simulink model "test_environment"  (R2019b)
settings: Solver=VariableStepAuto  StartTime=0.0  StopTime=100.0  FixedStep=1e-3  RelTol=1e-3
InitFcn:
  | data
undefined symbols (not defined in the file): __PRM__SERIALIZED__DATA__, juliandate, r, r_bo, RP, SubsystemReferenceBlock
libraries: simulink x4
settings Model: Creator=imanol  LastModifiedBy=imanol

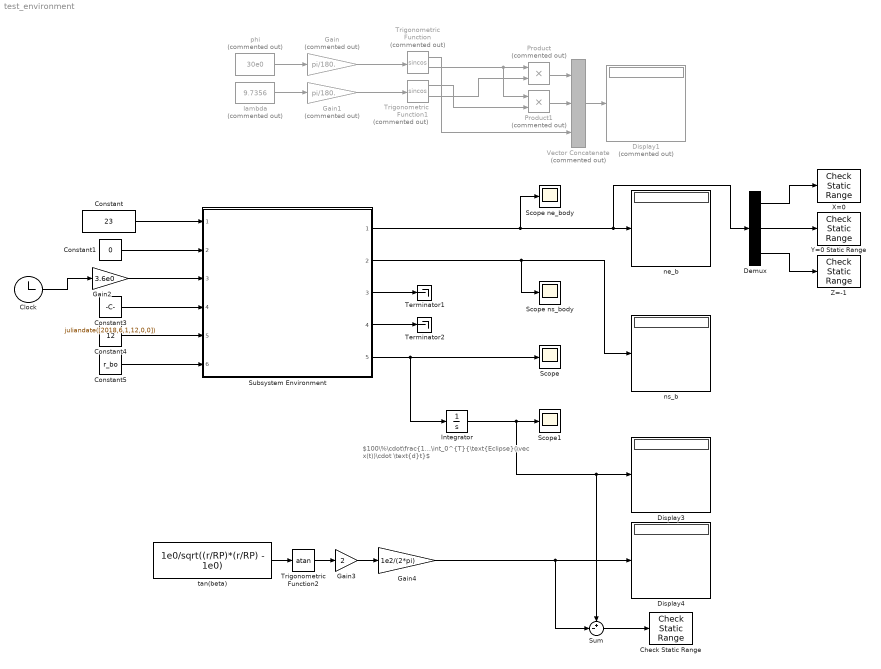
== system test_environment ==
  note: $100\%\cdot\frac{1}{T}\int_0^{T}{\text{Eclipse}(\vec x(t))\cdot \text{d}t}$
  Check Static Range : simulink/Model Verification/Check  Static Range  Description=-1e2 <= u <= 2e0  max=2e0  max_included=on  min=-1e2  min_included=on  enabled=on  stopWhenAssertionFail=on  export=off  icon=graphic
      settings: SourceProductName=Simulink  SourceProductBaseCode=SL
  Clock : Clock
      settings: Decimation=100
  Constant : Constant  Value=23
  Constant1 : Constant  Value=0
  Constant3 : Constant  Value=juliandate([2018,6,1,12,0,0])
  Constant4 : Constant  Value=12
  Constant5 : Constant  Value=r_bo
  Demux : Demux  Outputs=3
  Display1 : Display  Commented=on
  Display3 : Display
  Display4 : Display
  Gain : Gain  Commented=on  Gain=pi/180.
  Gain1 : Gain  Commented=on  Gain=pi/180.
  Gain2 : Gain  Gain=3.6e0
  Gain3 : Gain  Gain=2
  Gain4 : Gain  Gain=1e2/(2*pi)
  Integrator : Integrator  InitialCondition=0e0
  Product : Product  Commented=on
  Product1 : Product  Commented=on
  Scope : Scope
  Scope ne_body : Scope
  Scope ns_body : Scope
  Scope1 : Scope
  Subsystem Environment : Subsystem  BlockKeywords=__PRM__SERIALIZED__DATA__:SubsystemReferenceBlock  ReferencedSubsystem=block_environment
  Sum : Sum  Inputs=+-|
  Terminator1 : Terminator
  Terminator2 : Terminator
  Trigonometric Function : Trigonometry  Commented=on  Operator=sincos
  Trigonometric Function1 : Trigonometry  Commented=on  Operator=sincos
  Trigonometric Function2 : Trigonometry  Operator=atan
  Vector Concatenate : Concatenate  Commented=on  NumInputs=3
  X=0 : simulink/Model Verification/Check  Static Range  Description=0e0 - 1e-5 <= u <= 0e0 + 1e-5  max=0e0 + 1e-5  max_included=on  min=0e0 - 1e-5  min_included=on  enabled=on  stopWhenAssertionFail=on  export=off  icon=graphic
      settings: SourceProductName=Simulink  SourceProductBaseCode=SL
  Y=0 Static Range : simulink/Model Verification/Check  Static Range  Description=0e0 - 1e-5 <= u <= 0e0 + 1e-5  max=0e0 + 1e-5  max_included=on  min=0e0 - 1e-5  min_included=on  enabled=on  stopWhenAssertionFail=on  export=off  icon=graphic
      settings: SourceProductName=Simulink  SourceProductBaseCode=SL
  "Z=-1 " : simulink/Model Verification/Check  Static Range  Description=-1e0 - 1e-5 <= u <= -1e0 + 1e-5  max=-1e0 + 1e-5  max_included=on  min=-1e0 - 1e-5  min_included=on  enabled=on  stopWhenAssertionFail=on  export=off  icon=graphic
      settings: SourceProductName=Simulink  SourceProductBaseCode=SL
  lambda : Constant  Commented=on  Value=9.7356
  ne_b : Display
  ns_b : Display
  phi : Constant  Commented=on  Value=30e0
  tan(beta) : Constant  Value=1e0/sqrt((r/RP)*(r/RP) - 1e0)
  wires:
  Constant/1 -> Subsystem Environment/1
  Constant1/1 -> Subsystem Environment/2
  Gain2/1 -> Subsystem Environment/3
  Constant3/1 -> Subsystem Environment/4
  Constant4/1 -> Subsystem Environment/5
  Subsystem Environment/1 -> Scope ne_body/1, Demux/1, ne_b/1
  Subsystem Environment/4 -> Terminator2/1
  Subsystem Environment/3 -> Terminator1/1
  Subsystem Environment/2 -> ns_b/1, Scope ns_body/1
  Constant5/1 -> Subsystem Environment/6
  phi/1 -> Gain/1
  lambda/1 -> Gain1/1
  Gain1/1 -> Trigonometric Function1/1
  Gain/1 -> Trigonometric Function/1
  Trigonometric Function/2 -> Product1/1, Product/1
  Trigonometric Function1/2 -> Product/2
  Trigonometric Function1/1 -> Product1/2
  Product/1 -> Vector Concatenate/1
  Product1/1 -> Vector Concatenate/2
  Trigonometric Function/1 -> Vector Concatenate/3
  Vector Concatenate/1 -> Display1/1
  Clock/1 -> Gain2/1
  Integrator/1 -> Scope1/1, Sum/1, Display3/1
  Subsystem Environment/5 -> Integrator/1, Scope/1
  Demux/2 -> Y=0 Static Range/1
  Demux/1 -> X=0/1
  Demux/3 -> "Z=-1 "/1
  Gain4/1 -> Sum/2, Display4/1
  Sum/1 -> Check Static Range/1
  tan(beta)/1 -> Trigonometric Function2/1
  Trigonometric Function2/1 -> Gain3/1
  Gain3/1 -> Gain4/1
